simulink model "MRC_demo"  (Simulink 7.6)
settings: Solver=ode45  StartTime=0.0  StopTime=inf  RelTol=1e-3
libraries: commchan3 x8, commdigbbndpm3 x2, commrandsrc2 x1, commsink2 x1
settings Model: Creator=Administrator  LastModifiedBy=Administrator

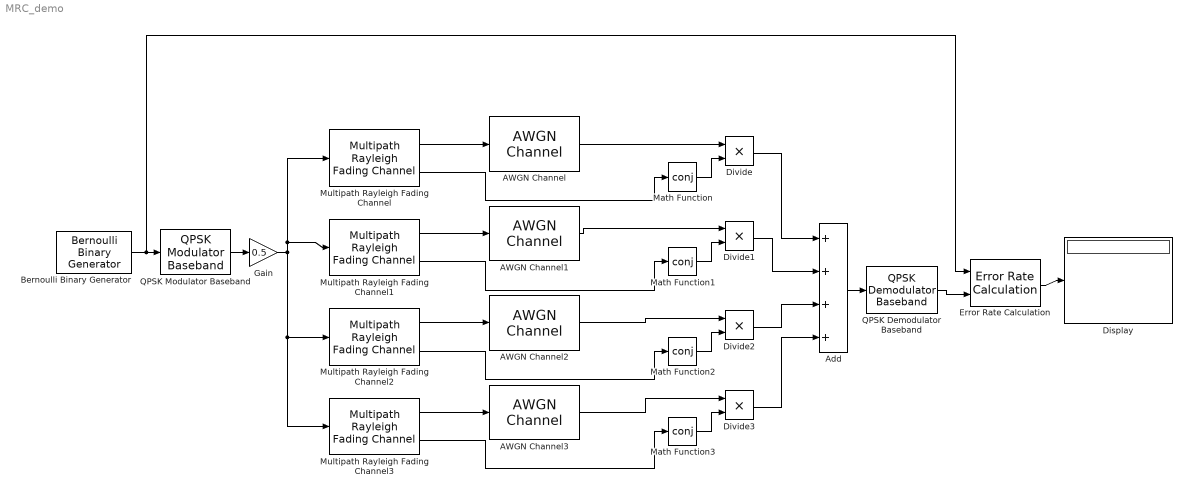
== system MRC_demo ==
  AWGN Channel : commchan3/AWGN Channel  SystemSampleTime=-1  InputProcessing=Columns as channels (frame based)  seed=67  noiseMode="Signal to noise ratio  (Eb/No)"  EbNodB=10  EsNodB=10  SNRdB=10  bitsPerSym=2  Ps=1  Tsym=1e-3  variance=1
  AWGN Channel1 : commchan3/AWGN Channel  SystemSampleTime=-1  InputProcessing=Columns as channels (frame based)  seed=671  noiseMode="Signal to noise ratio  (Eb/No)"  EbNodB=10  EsNodB=10  SNRdB=10  bitsPerSym=2  Ps=1  Tsym=1e-3  variance=1
  AWGN Channel2 : commchan3/AWGN Channel  SystemSampleTime=-1  InputProcessing=Columns as channels (frame based)  seed=6711  noiseMode="Signal to noise ratio  (Eb/No)"  EbNodB=10  EsNodB=10  SNRdB=10  bitsPerSym=2  Ps=1  Tsym=1e-3  variance=1
  AWGN Channel3 : commchan3/AWGN Channel  SystemSampleTime=-1  InputProcessing=Columns as channels (frame based)  seed=67111  noiseMode="Signal to noise ratio  (Eb/No)"  EbNodB=10  EsNodB=10  SNRdB=10  bitsPerSym=2  Ps=1  Tsym=1e-3  variance=1
  Add : Sum  Inputs=++++
  Bernoulli Binary Generator : commrandsrc2/Bernoulli Binary Generator  DialogController=commDDGCreate  DialogControllerArgs=DataTag4  SystemSampleTime=-1  P=0.5  seed=61  Ts=0.5e-3  frameBased=on  sampPerFrame=100  orient=off  outDataType=double
  Display : Display
  Divide{,1..3} (4 alike) : Product  Inputs=**
  Error Rate Calculation : commsink2/Error Rate Calculation  N=0  st_delay=0  cp_mode=Entire frame  subframe=[]  PMode=Port  WsName=ErrorVec  RsMode2=off  stop=off  numErr=100  maxBits=1e6
  Gain : Gain  Gain=0.5
  Math Function{,1..3} (4 alike) : Math  Operator=conj  SaturateOnIntegerOverflow=on
  Multipath Rayleigh Fading Channel : commchan3/Multipath Rayleigh Fading Channel  SystemSampleTime=-1  maxDopplerShift=40  spectrumType=Jakes  sigmaGaussian=1/sqrt(2)  coeffRounded=[1 -1.72 0.785]  freqMinMaxRJakes=[0 1]  freqMinMaxAJakes=[0 1]  sigmaGaussian1=1/sqrt(2)  sigmaGaussian2=1/sqrt(2)  centerFreqGaussian1=0.0  centerFreqGaussian2=0.0  gainGaussian1=0.5  gainGaussian2=0.5  coeffBell=9  dopplerSpectrum=doppler.jakes  pathDelays=0  avgPathGaindB=0  normalizePathGains=on  seed=73  enableProbe=0  openVisAtStart=off  outPathGains=on  outDelay=off
  Multipath Rayleigh Fading Channel1 : commchan3/Multipath Rayleigh Fading Channel  SystemSampleTime=-1  maxDopplerShift=40  spectrumType=Jakes  sigmaGaussian=1/sqrt(2)  coeffRounded=[1 -1.72 0.785]  freqMinMaxRJakes=[0 1]  freqMinMaxAJakes=[0 1]  sigmaGaussian1=1/sqrt(2)  sigmaGaussian2=1/sqrt(2)  centerFreqGaussian1=0.0  centerFreqGaussian2=0.0  gainGaussian1=0.5  gainGaussian2=0.5  coeffBell=9  dopplerSpectrum=doppler.jakes  pathDelays=0  avgPathGaindB=0  normalizePathGains=on  seed=731  enableProbe=0  openVisAtStart=off  outPathGains=on  outDelay=off
  Multipath Rayleigh Fading Channel2 : commchan3/Multipath Rayleigh Fading Channel  SystemSampleTime=-1  maxDopplerShift=40  spectrumType=Jakes  sigmaGaussian=1/sqrt(2)  coeffRounded=[1 -1.72 0.785]  freqMinMaxRJakes=[0 1]  freqMinMaxAJakes=[0 1]  sigmaGaussian1=1/sqrt(2)  sigmaGaussian2=1/sqrt(2)  centerFreqGaussian1=0.0  centerFreqGaussian2=0.0  gainGaussian1=0.5  gainGaussian2=0.5  coeffBell=9  dopplerSpectrum=doppler.jakes  pathDelays=0  avgPathGaindB=0  normalizePathGains=on  seed=7311  enableProbe=0  openVisAtStart=off  outPathGains=on  outDelay=off
  Multipath Rayleigh Fading Channel3 : commchan3/Multipath Rayleigh Fading Channel  SystemSampleTime=-1  maxDopplerShift=40  spectrumType=Jakes  sigmaGaussian=1/sqrt(2)  coeffRounded=[1 -1.72 0.785]  freqMinMaxRJakes=[0 1]  freqMinMaxAJakes=[0 1]  sigmaGaussian1=1/sqrt(2)  sigmaGaussian2=1/sqrt(2)  centerFreqGaussian1=0.0  centerFreqGaussian2=0.0  gainGaussian1=0.5  gainGaussian2=0.5  coeffBell=9  dopplerSpectrum=doppler.jakes  pathDelays=0  avgPathGaindB=0  normalizePathGains=on  seed=73111  enableProbe=0  openVisAtStart=off  outPathGains=on  outDelay=off
  QPSK Demodulator Baseband : commdigbbndpm3/QPSK Demodulator Baseband  DialogController=commDDGCreate  DialogControllerArgs=DataTag5  Ph=pi/4  Dec=Gray  OutType=Bit  DecType=Hard decision  VarSource=Dialog  Variance=1  outDtype1=Inherit via internal rule  outDtype2=Inherit via internal rule  derotateFactorWordLen=16
  QPSK Modulator Baseband : commdigbbndpm3/QPSK Modulator Baseband  DialogController=commDDGCreate  DialogControllerArgs=DataTag6  SystemSampleTime=-1  InType=Bit  Enc=Gray  Ph=pi/4  outDtype=double  outWordLen=16  outUDDataType=sfix(16)  outFracLenMode=Best precision  outFracLen=15
  wires:
  Bernoulli Binary Generator/1 -> QPSK Modulator Baseband/1, Error Rate Calculation/1
  QPSK Modulator Baseband/1 -> Gain/1
  Multipath Rayleigh Fading Channel/1 -> AWGN Channel/1
  Multipath Rayleigh Fading Channel1/1 -> AWGN Channel1/1
  Multipath Rayleigh Fading Channel2/1 -> AWGN Channel2/1
  Multipath Rayleigh Fading Channel3/1 -> AWGN Channel3/1
  AWGN Channel/1 -> Divide/1
  Math Function/1 -> Divide/2
  Multipath Rayleigh Fading Channel/2 -> Math Function/1
  AWGN Channel1/1 -> Divide1/1
  Math Function1/1 -> Divide1/2
  Math Function2/1 -> Divide2/2
  Math Function3/1 -> Divide3/2
  AWGN Channel2/1 -> Divide2/1
  AWGN Channel3/1 -> Divide3/1
  Multipath Rayleigh Fading Channel1/2 -> Math Function1/1
  Multipath Rayleigh Fading Channel3/2 -> Math Function3/1
  Multipath Rayleigh Fading Channel2/2 -> Math Function2/1
  Divide/1 -> Add/1
  Divide1/1 -> Add/2
  Divide2/1 -> Add/3
  Divide3/1 -> Add/4
  Add/1 -> QPSK Demodulator Baseband/1
  Error Rate Calculation/1 -> Display/1
  QPSK Demodulator Baseband/1 -> Error Rate Calculation/2
  Gain/1 -> Multipath Rayleigh Fading Channel/1, Multipath Rayleigh Fading Channel1/1, Multipath Rayleigh Fading Channel3/1, Multipath Rayleigh Fading Channel2/1
